simulink model "model3"  (Simulink 6.5)
settings: Solver=ode4  SolverMode=SingleTasking  StartTime=0.0  StopTime=10.0  FixedStep=1e-2  RelTol=1e-3
undefined symbols (not defined in the file): A, AP, B, BP, C, CP, D, H, WPC
settings Model: Creator=bartek  LastModifiedBy=bartek
settings DataIOCC: LimitDataPoints=off
settings OptimizationCC: InitFltsAndDblsToZero=off
settings DebuggingCC: SignalResolutionControl=UseLocalSettings
settings HardwareCC: TargetHWDeviceType=32-bit Generic
settings GRTTargetCC: ExtModeInterfaceLevel=Level1

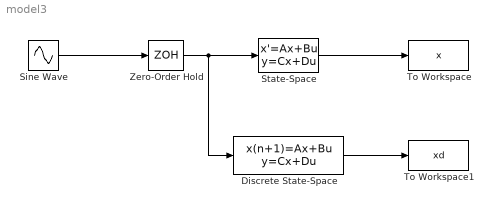
== system model3 ==
  Discrete State-Space : DiscreteStateSpace  A=AP  B=BP  C=CP  D=D  X0=WPC  SampleTime=H
  Sine Wave : Sin  Amplitude=1  Bias=0  Frequency=1  Phase=0  Samples=10  Offset=0
  State-Space : StateSpace  A=A  B=B  C=C  D=D  X0=WPC
  To Workspace : ToWorkspace  VariableName=x  SampleTime=1E-2  SaveFormat=Array
  To Workspace1 : ToWorkspace  VariableName=xd  SampleTime=1e-2  SaveFormat=Array
  Zero-Order Hold : ZeroOrderHold  SampleTime=H
  wires:
  Zero-Order Hold/1 -> State-Space/1, Discrete State-Space/1
  State-Space/1 -> To Workspace/1
  Discrete State-Space/1 -> To Workspace1/1
  Sine Wave/1 -> Zero-Order Hold/1
